simulink model "Practica_4"  (R2022b)
settings: Solver=VariableStepAuto  StartTime=0.0  StopTime=10.0  RelTol=1e-3
values from neighbouring files (symbols this model uses):
  k = 100    [KPMC.m]    (also in Parametros_Practica_4.m)
  m = 10    [KPMC.m]    (also in Parametros_Practica_4.m)
settings Model: Creator=escor  LastModifiedBy=escor

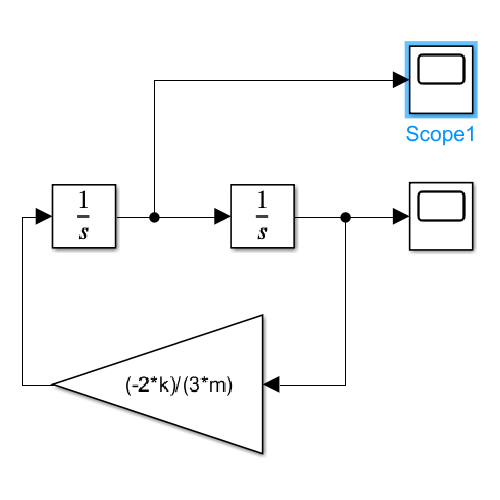
[thumbnail: Simulink's stored preview of the top-level diagram]
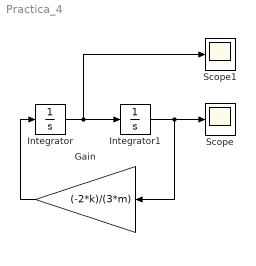
== system Practica_4 ==
  Gain : Gain  Gain=(-2*k)/(3*m)
  Integrator : Integrator  InitialCondition=2
  Integrator1 : Integrator
  Scope : Scope
  Scope1 : Scope
  wires:
  Integrator/1 -> Scope1/1, Integrator1/1
  Gain/1 -> Integrator/1
  Integrator1/1 -> Scope/1, Gain/1
